simulink model "CrossCorrelator_q"  (R2018b)
settings: Solver=FixedStepAuto  StartTime=0.0  StopTime=500*(15e-9)  FixedStep=15e-9  RelTol=1e-3
libraries: hdlsllib x14, simulink x8
settings Model: Creator=meyer  LastModifiedBy=meyer
settings OptimizationCC: DefaultParameterBehavior=Inlined

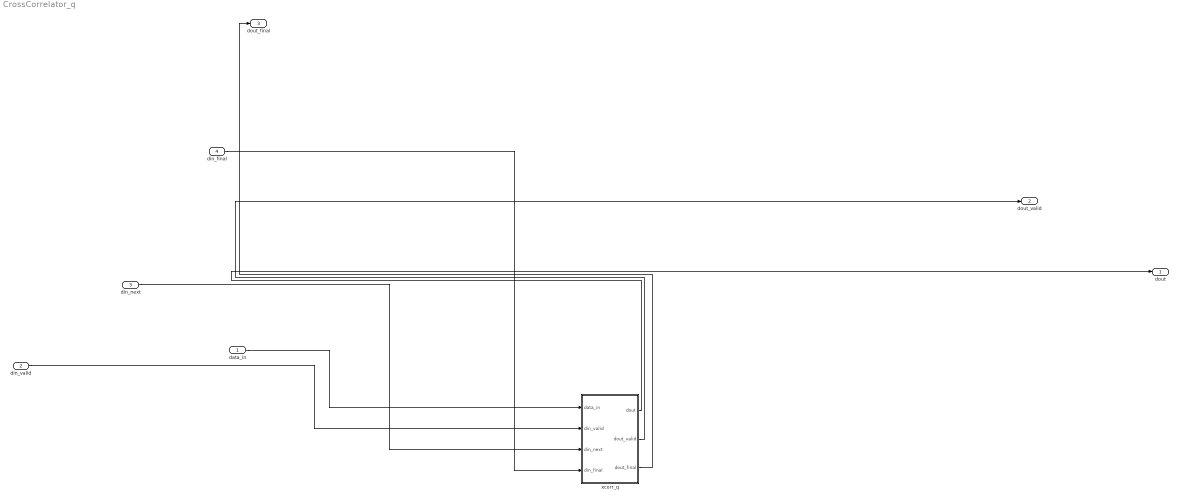
== system CrossCorrelator_q ==
  data_in : Inport  OutDataTypeStr=fixdt(1,16,15)
  din_valid : Inport  Port=2
  din_next : Inport  Port=3
  din_final : Inport  Port=4
  xcorr_q : Subsystem
  dout : Outport  OutDataTypeStr=fixdt(1,32,16)
  dout_valid : Outport  Port=2
  dout_final : Outport  Port=3
  wires:
  data_in/1 -> xcorr_q/1(data_in)
  din_valid/1 -> xcorr_q/2(din_valid)
  din_next/1 -> xcorr_q/3(din_next)
  din_final/1 -> xcorr_q/4(din_final)
  xcorr_q/1(dout) -> dout/1
  xcorr_q/2(dout_valid) -> dout_valid/1
  xcorr_q/3(dout_final) -> dout_final/1

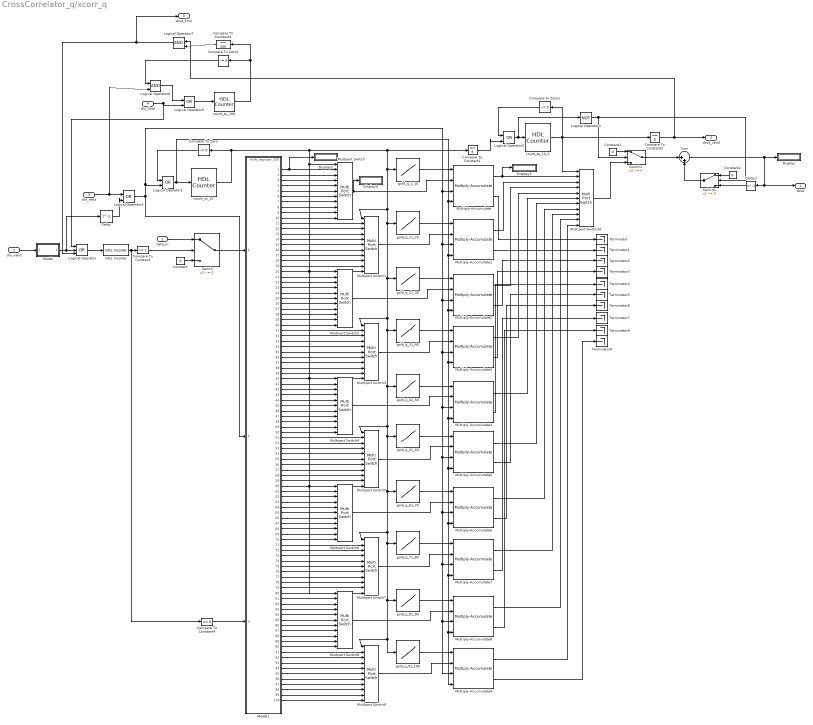
== system CrossCorrelator_q/xcorr_q ==
  data_in : Inport  OutDataTypeStr=fixdt(1,16,15)
  din_valid : Inport  Port=2
  din_next : Inport  Port=3
  din_final : Inport  Port=4
  Compare To Constant : simulink/Logic and Bit Operations/Compare To Constant  relop===  const=1  OutDataTypeStr=boolean
  Compare To Constant1 : simulink/Logic and Bit Operations/Compare To Constant  relop===  const=9  OutDataTypeStr=boolean
  Compare To Constant2 : simulink/Logic and Bit Operations/Compare To Constant  relop===  const=9  OutDataTypeStr=boolean
  Compare To Constant3 : simulink/Logic and Bit Operations/Compare To Constant  relop===  const=100  OutDataTypeStr=boolean
  Compare To Constant4 : simulink/Logic and Bit Operations/Compare To Constant  relop===  const=0  OutDataTypeStr=boolean
  Compare To Zero : simulink/Logic and Bit Operations/Compare To Zero  relop=~=  OutDataTypeStr=boolean
  Compare To Zero1 : simulink/Logic and Bit Operations/Compare To Zero  relop=~=  OutDataTypeStr=boolean
  Compare To Zero2 : simulink/Logic and Bit Operations/Compare To Zero  relop=~=  OutDataTypeStr=boolean
  Constant : Constant  Value=0  OutDataTypeStr=fixdt(1,16,15)  SampleTime=-1
  Constant1 : Constant  Value=0  OutDataTypeStr=Inherit: Inherit via back propagation  SampleTime=-1
  Constant2 : Constant  Value=0  OutDataTypeStr=Inherit: Inherit via back propagation  SampleTime=-1
  Delay : Delay  DelayLength=1
  Delay1 : Delay  DelayLength=1
  Display{,1..3} (4 alike) : Display
  HDL Counter : hdlsllib/Sources/HDL Counter  CountType=Count limited  CountInit=0  CountStep=1  CountMax=2  CountFromType=Initial value  CountFrom=0  CountResetPort=off  CountLoadPort=off  CountEnbPort=on  CountDirPort=off  CountDataType=Unsigned  CountWordLen=8  CountFracLen=0  CountSampTime=1
      settings: SourceProductBaseCode=HD
  Logical Operator : Logic  Operator=OR  Inputs=3  IconShape=distinctive  AllPortsSameDT=off  OutDataTypeStr=boolean
  Logical Operator{1..3,5} (4 alike) : Logic  Operator=OR  IconShape=distinctive  AllPortsSameDT=off  OutDataTypeStr=boolean
  Logical Operator4 : Logic  Operator=NOT  IconShape=distinctive  AllPortsSameDT=off  OutDataTypeStr=boolean
  Logical Operator6 : Logic  IconShape=distinctive  AllPortsSameDT=off  OutDataTypeStr=boolean
  Logical Operator7 : Logic  IconShape=distinctive  AllPortsSameDT=off  OutDataTypeStr=boolean
  Model : ModelReference  ModelNameDialog=re_detect  SimulationMode=Normal  ModelReferenceVersion=1.7
  Model1 : ModelReference  ModelNameDialog=shift_register_100  SimulationMode=Normal  ModelReferenceVersion=1.17
  Multiply-Accumulate{,1..9} (10 alike) : hdlsllib/HDL Operations/Multiply-Accumulate  opMode=Streaming - using Start and End ports  initValueSetting=Dialog  initValue=0  initValueSetting2=Dialog  initValue2=0  initValueSetting3=Dialog  initValue3=0  num_samples=2  RndMeth2=Floor  RndMeth3=Floor  datatype2=fixdt(1,32,16)  datatype3=Inherit: Inherit via back propagation  validOut=on  endInandOut=off  startOut=off  countOut=on  dim=-1  DoSatur=off  parallel=off
      settings: SourceProductName=HDL Coder  SourceProductBaseCode=HD
  Multiport Switch{,1..9} (10 alike) : MultiPortSwitch  DataPortOrder=Zero-based contiguous  Inputs=10  zeroidx=on  OutDataTypeStr=fixdt(1,16,15)
  Multiport Switch10 : MultiPortSwitch  DataPortOrder=Zero-based contiguous  Inputs=10  zeroidx=on  OutDataTypeStr=fixdt(1,32,16)
  Sum : Sum  Inputs=|++  OutDataTypeStr=Inherit: Inherit via back propagation
  Switch : Switch  Criteria=u2 ~= 0  OutDataTypeStr=Inherit: Inherit via back propagation
  Switch1 : Switch  Criteria=u2 ~= 0  OutDataTypeStr=Inherit: Inherit via back propagation
  Switch2 : Switch  Criteria=u2 ~= 0  OutDataTypeStr=Inherit: Inherit via back propagation
  Terminator{,1..9} (10 alike) : Terminator
  count_to_10 : hdlsllib/Sources/HDL Counter  CountType=Count limited  CountInit=0  CountStep=1  CountMax=9  CountFromType=Initial value  CountFrom=0  CountResetPort=off  CountLoadPort=off  CountEnbPort=on  CountDirPort=off  CountDataType=Unsigned  CountWordLen=4  CountFracLen=0  CountSampTime=1
      settings: SourceProductBaseCode=HD
  count_to_100 : hdlsllib/Sources/HDL Counter  CountType=Count limited  CountInit=0  CountStep=1  CountMax=100  CountFromType=Initial value  CountFrom=0  CountResetPort=off  CountLoadPort=off  CountEnbPort=on  CountDirPort=off  CountDataType=Unsigned  CountWordLen=8  CountFracLen=0  CountSampTime=1
      settings: SourceProductBaseCode=HD
  count_to_10_2 : hdlsllib/Sources/HDL Counter  CountType=Count limited  CountInit=0  CountStep=1  CountMax=9  CountFromType=Initial value  CountFrom=0  CountResetPort=off  CountLoadPort=off  CountEnbPort=on  CountDirPort=off  CountDataType=Unsigned  CountWordLen=4  CountFracLen=0  CountSampTime=1
      settings: SourceProductBaseCode=HD
  gold_q_11_20 : Lookup_n-D  NumberOfTableDimensions=1  LookupTableObject=''  BreakpointsForDimension1=uint8([0,1,2,3,4,5,6,7,8,9])  BreakpointsForDimension1FirstPoint=10  BreakpointsForDimension2FirstPoint=10  BreakpointsForDimension1Spacing=12  BreakpointsForDimension2Spacing=12  IndexSearchMethod=Evenly spaced points  Table=|  TableDataTypeStr=fixdt(1,16,15)  InterpMethod=Flat  DiagnosticForOutOfRangeInput=Error  InternalRulePriority=Speed  OutDataTypeStr=fixdt(1,16,15)  RndMeth=Simplest  InputSameDT=on
      | -1*[0.236906374990369
      | 0.265062589296935
      | 0.290853922757751
      | 0.306866645010829
      | 0.306877356493505
      | 0.282583044796408
      | 0.237895318583737
      | 0.179451570247324
      | 0.106711739895776
      | 0.0250742736874029]
  gold_q_1_10 : Lookup_n-D  NumberOfTableDimensions=1  LookupTableObject=''  BreakpointsForDimension1=uint8([0,1,2,3,4,5,6,7,8,9])  BreakpointsForDimension1FirstPoint=10  BreakpointsForDimension2FirstPoint=10  BreakpointsForDimension1Spacing=12  BreakpointsForDimension2Spacing=12  IndexSearchMethod=Evenly spaced points  Table=|  TableDataTypeStr=fixdt(1,16,15)  InterpMethod=Flat  DiagnosticForOutOfRangeInput=Error  InternalRulePriority=Speed  OutDataTypeStr=fixdt(1,16,15)  RndMeth=Simplest  InputSameDT=on
      | -1*[0.357169275362262
      | 0.373691122276015
      | 0.363136475782144
      | 0.332586509539436
      | 0.291374087870011
      | 0.249422279627694
      | 0.215579045674242
      | 0.200455944131647
      | 0.201796906991478
      | 0.213779029408702]
  gold_q_21_30 : Lookup_n-D  NumberOfTableDimensions=1  LookupTableObject=''  BreakpointsForDimension1=uint8([0,1,2,3,4,5,6,7,8,9])  BreakpointsForDimension1FirstPoint=10  BreakpointsForDimension2FirstPoint=10  BreakpointsForDimension1Spacing=12  BreakpointsForDimension2Spacing=12  IndexSearchMethod=Evenly spaced points  Table=|  TableDataTypeStr=fixdt(1,16,15)  InterpMethod=Flat  DiagnosticForOutOfRangeInput=Error  InternalRulePriority=Speed  OutDataTypeStr=fixdt(1,16,15)  RndMeth=Simplest  InputSameDT=on
      | -1*[-0.0591515848508664
      | -0.139598314313151
      | -0.210629837752387
      | -0.263713716480122
      | -0.301489962058033
      | -0.328238114626508
      | -0.340130412877520
      | -0.338689881672749
      | -0.326243180584237
      | -0.305614110780615]
  gold_q_31_40 : Lookup_n-D  NumberOfTableDimensions=1  LookupTableObject=''  BreakpointsForDimension1=uint8([0,1,2,3,4,5,6,7,8,9])  BreakpointsForDimension1FirstPoint=10  BreakpointsForDimension2FirstPoint=10  BreakpointsForDimension1Spacing=12  BreakpointsForDimension2Spacing=12  IndexSearchMethod=Evenly spaced points  Table=|  TableDataTypeStr=fixdt(1,16,15)  InterpMethod=Flat  DiagnosticForOutOfRangeInput=Error  InternalRulePriority=Speed  OutDataTypeStr=fixdt(1,16,15)  RndMeth=Simplest  InputSameDT=on
      | -1*[-0.279858098355888
      | -0.247814863771713
      | -0.225446174923891
      | -0.202743193363060
      | -0.186527042991191
      | -0.178781266249413
      | -0.180711431323688
      | -0.192575241083779
      | -0.213551675353351
      | -0.245925394077466]
  gold_q_41_50 : Lookup_n-D  NumberOfTableDimensions=1  LookupTableObject=''  BreakpointsForDimension1=uint8([0,1,2,3,4,5,6,7,8,9])  BreakpointsForDimension1FirstPoint=10  BreakpointsForDimension2FirstPoint=10  BreakpointsForDimension1Spacing=12  BreakpointsForDimension2Spacing=12  IndexSearchMethod=Evenly spaced points  Table=|  TableDataTypeStr=fixdt(1,16,15)  InterpMethod=Flat  DiagnosticForOutOfRangeInput=Error  InternalRulePriority=Speed  OutDataTypeStr=fixdt(1,16,15)  RndMeth=Simplest  InputSameDT=on
      | -1*[-0.273649789754997
      | -0.305507933389466
      | -0.332526349511340
      | -0.349961882407133
      | -0.353614169955030
      | -0.340366684130075
      | -0.308641627170326
      | -0.254460428744123
      | -0.185247665828561
      | -0.110080691949015]
  gold_q_51_60 : Lookup_n-D  NumberOfTableDimensions=1  LookupTableObject=''  BreakpointsForDimension1=uint8([0,1,2,3,4,5,6,7,8,9])  BreakpointsForDimension1FirstPoint=10  BreakpointsForDimension2FirstPoint=10  BreakpointsForDimension1Spacing=12  BreakpointsForDimension2Spacing=12  IndexSearchMethod=Evenly spaced points  Table=|  TableDataTypeStr=fixdt(1,16,15)  InterpMethod=Flat  DiagnosticForOutOfRangeInput=Error  InternalRulePriority=Speed  OutDataTypeStr=fixdt(1,16,15)  RndMeth=Simplest  InputSameDT=on
      | -1*[-0.0297558495000079
      | 0.0499350486257353
      | 0.122950591883728
      | 0.183532283875116
      | 0.226715241693549
      | 0.244522518247979
      | 0.247772413924009
      | 0.223279362418140
      | 0.176793915855740
      | 0.111355596734925]
  gold_q_61_70 : Lookup_n-D  NumberOfTableDimensions=1  LookupTableObject=''  BreakpointsForDimension1=uint8([0,1,2,3,4,5,6,7,8,9])  BreakpointsForDimension1FirstPoint=10  BreakpointsForDimension2FirstPoint=10  BreakpointsForDimension1Spacing=12  BreakpointsForDimension2Spacing=12  IndexSearchMethod=Evenly spaced points  Table=|  TableDataTypeStr=fixdt(1,16,15)  InterpMethod=Flat  DiagnosticForOutOfRangeInput=Error  InternalRulePriority=Speed  OutDataTypeStr=fixdt(1,16,15)  RndMeth=Simplest  InputSameDT=on
      | -1*[0.0312880626224120
      | -0.0580988665112754
      | -0.150830519884918
      | -0.236354458852815
      | -0.321361371110983
      | -0.387151947785857
      | -0.432910784333285
      | -0.454553321854592
      | -0.449340647995131
      | -0.416266380216616]
  gold_q_71_80 : Lookup_n-D  NumberOfTableDimensions=1  LookupTableObject=''  BreakpointsForDimension1=uint8([0,1,2,3,4,5,6,7,8,9])  BreakpointsForDimension1FirstPoint=10  BreakpointsForDimension2FirstPoint=10  BreakpointsForDimension1Spacing=12  BreakpointsForDimension2Spacing=12  IndexSearchMethod=Evenly spaced points  Table=|  TableDataTypeStr=fixdt(1,16,15)  InterpMethod=Flat  DiagnosticForOutOfRangeInput=Error  InternalRulePriority=Speed  OutDataTypeStr=fixdt(1,16,15)  RndMeth=Simplest  InputSameDT=on
      | -1*[-0.356405677154333
      | -0.268905527196357
      | -0.172503144328213
      | -0.0623088722264564
      | 0.0478292512438748
      | 0.147701871156711
      | 0.227579808283800
      | 0.279365016179912
      | 0.297653875710056
      | 0.276310228166542]
  gold_q_81_90 : Lookup_n-D  NumberOfTableDimensions=1  LookupTableObject=''  BreakpointsForDimension1=uint8([0,1,2,3,4,5,6,7,8,9])  BreakpointsForDimension1FirstPoint=10  BreakpointsForDimension2FirstPoint=10  BreakpointsForDimension1Spacing=12  BreakpointsForDimension2Spacing=12  IndexSearchMethod=Evenly spaced points  Table=|  TableDataTypeStr=fixdt(1,16,15)  InterpMethod=Flat  DiagnosticForOutOfRangeInput=Error  InternalRulePriority=Speed  OutDataTypeStr=fixdt(1,16,15)  RndMeth=Simplest  InputSameDT=on
      | -1*[0.222595237130309
      | 0.147485843722747
      | 0.0555170073150737
      | -0.0424496465550990
      | -0.134707118174198
      | -0.210100315272752
      | -0.259403813850479
      | -0.272248751146779
      | -0.259403813850479
      | -0.210100315272752]
  gold_q_91_100 : Lookup_n-D  NumberOfTableDimensions=1  LookupTableObject=''  BreakpointsForDimension1=uint8([0,1,2,3,4,5,6,7,8,9])  BreakpointsForDimension1FirstPoint=10  BreakpointsForDimension2FirstPoint=10  BreakpointsForDimension1Spacing=12  BreakpointsForDimension2Spacing=12  IndexSearchMethod=Evenly spaced points  Table=|  TableDataTypeStr=fixdt(1,16,15)  InterpMethod=Flat  DiagnosticForOutOfRangeInput=Error  InternalRulePriority=Speed  OutDataTypeStr=fixdt(1,16,15)  RndMeth=Simplest  InputSameDT=on
      | -1*[-0.134707118174198
      | -0.0424496465550989
      | 0.0555170073150737
      | 0.147485843722747
      | 0.222595237130309
      | 0.267820298855522
      | 0.290378842162360
      | 0.275261187855880
      | 0.228204197191429
      | 0.153805243290024]
  dout : Outport  OutDataTypeStr=fixdt(1,32,16)
  dout_valid : Outport  Port=2
  dout_final : Outport  Port=3
  wires:
  Model1/63 -> Multiport Switch6/4
  Model1/83 -> Multiport Switch8/4
  Model1/87 -> Multiport Switch8/8
  Model1/57 -> Multiport Switch5/8
  count_to_10/1 -> Compare To Zero/1, Multiport Switch8/1, Multiport Switch6/1, Multiport Switch4/1, Multiport Switch2/1, Multiport Switch/1, gold_q_11_20/1, gold_q_21_30/1, gold_q_31_40/1, gold_q_41_50/1, gold_q_51_60/1, gold_q_61_70/1, gold_q_71_80/1, gold_q_81_90/1, gold_q_91_100/1, Multiport Switch9/1, Multiport Switch7/1, Multiport Switch5/1, Multiport Switch3/1, Multiport Switch1/1, gold_q_1_10/1, Compare To Constant1/1
  Model1/97 -> Multiport Switch9/8
  Multiply-Accumulate4/1 -> Multiport Switch10/6
  Model1/65 -> Multiport Switch6/6
  Model1/99 -> Multiport Switch9/10
  Model1/73 -> Multiport Switch7/4
  Model1/49 -> Multiport Switch4/10
  Multiply-Accumulate/2 -> Terminator/1
  din_final/1 -> Logical Operator/1, Logical Operator5/2
  count_to_10_2/1 -> Compare To Constant2/1, Multiport Switch10/1, Compare To Zero1/1
  Multiport Switch8/1 -> Multiply-Accumulate8/2
  Compare To Constant2/1 -> dout_valid/1, Logical Operator7/1
  Model1/61 -> Multiport Switch6/2
  Model1/28 -> Multiport Switch2/9
  Model1/1 -> Display2/1, Multiport Switch/2
  Multiply-Accumulate6/1 -> Multiport Switch10/8
  Model1/100 -> Multiport Switch9/11
  Logical Operator/1 -> HDL Counter/1
  din_valid/1 -> Model/1
  Model1/68 -> Multiport Switch6/9
  Model1/56 -> Multiport Switch5/7
  Model1/13 -> Multiport Switch1/4
  Model1/67 -> Multiport Switch6/8
  Model1/66 -> Multiport Switch6/7
  Logical Operator2/1 -> Logical Operator4/1, count_to_10_2/1
  Constant/1 -> Switch/3
  Compare To Zero/1 -> Logical Operator1/1
  Model1/89 -> Multiport Switch8/10
  Multiport Switch5/1 -> Multiply-Accumulate5/2
  Model1/29 -> Multiport Switch2/10
  Compare To Constant/1 -> Switch/2
  gold_q_91_100/1 -> Multiply-Accumulate9/1
  Model1/52 -> Multiport Switch5/3
  Model/1 -> Delay/1, Logical Operator/2
  Logical Operator1/1 -> count_to_10/1, Multiply-Accumulate2/4, Multiply-Accumulate9/4, Multiply-Accumulate8/4, Multiply-Accumulate7/4, Multiply-Accumulate6/4, Multiply-Accumulate5/4, Multiply-Accumulate4/4, Multiply-Accumulate3/4, Multiply-Accumulate1/4, Multiply-Accumulate/4
  Model1/76 -> Multiport Switch7/7
  Sum/1 -> dout/1, Delay1/1, Display/1
  Logical Operator3/1 -> Multiply-Accumulate9/3, Multiply-Accumulate8/3, Multiply-Accumulate7/3, Multiply-Accumulate6/3, Multiply-Accumulate5/3, Multiply-Accumulate4/3, Multiply-Accumulate3/3, Multiply-Accumulate2/3, Multiply-Accumulate1/3, Multiply-Accumulate/3, Logical Operator1/2, Model1/2
  Model1/2 -> Multiport Switch/3
  Model1/88 -> Multiport Switch8/9
  Model1/64 -> Multiport Switch6/5
  Model1/41 -> Multiport Switch4/2
  Multiply-Accumulate9/2 -> Terminator9/1
  din_next/1 -> Logical Operator6/2, Logical Operator3/1
  Model1/11 -> Multiport Switch1/2
  Model1/96 -> Multiport Switch9/7
  Switch1/1 -> Sum/1
  Model1/80 -> Multiport Switch7/11
  Model1/54 -> Multiport Switch5/5
  Model1/82 -> Multiport Switch8/3
  Multiply-Accumulate4/2 -> Terminator4/1
  Model1/6 -> Multiport Switch/7
  Model1/45 -> Multiport Switch4/6
  Multiport Switch4/1 -> Multiply-Accumulate4/2
  Logical Operator4/1 -> Switch1/2, Switch2/2
  Model1/58 -> Multiport Switch5/9
  Model1/81 -> Multiport Switch8/2
  Model1/44 -> Multiport Switch4/5
  Model1/86 -> Multiport Switch8/7
  Model1/85 -> Multiport Switch8/6
  Logical Operator5/1 -> count_to_100/1
  Multiport Switch/1 -> Multiply-Accumulate/2, Display3/1
  Model1/27 -> Multiport Switch2/8
  gold_q_31_40/1 -> Multiply-Accumulate3/1
  Model1/93 -> Multiport Switch9/4
  Compare To Zero1/1 -> Logical Operator2/1
  Model1/39 -> Multiport Switch3/10
  Model1/84 -> Multiport Switch8/5
  Model1/70 -> Multiport Switch6/11
  Model1/77 -> Multiport Switch7/8
  Model1/62 -> Multiport Switch6/3
  Model1/95 -> Multiport Switch9/6
  gold_q_1_10/1 -> Multiply-Accumulate/1
  Compare To Zero2/1 -> Logical Operator6/1
  Multiply-Accumulate1/1 -> Multiport Switch10/3
  Model1/47 -> Multiport Switch4/8
  Multiply-Accumulate3/2 -> Terminator3/1
  Model1/22 -> Multiport Switch2/3
  Model1/92 -> Multiport Switch9/3
  count_to_100/1 -> Compare To Constant3/1, Compare To Zero2/1
  Multiport Switch3/1 -> Multiply-Accumulate3/2
  Model1/59 -> Multiport Switch5/10
  Model1/9 -> Multiport Switch/10
  Model1/5 -> Multiport Switch/6
  gold_q_11_20/1 -> Multiply-Accumulate1/1
  data_in/1 -> Switch/1
  Model1/90 -> Multiport Switch8/11
  Model1/10 -> Multiport Switch/11
  Model1/75 -> Multiport Switch7/6
  Model1/18 -> Multiport Switch1/9
  Model1/12 -> Multiport Switch1/3
  Model1/25 -> Multiport Switch2/6
  Model1/43 -> Multiport Switch4/4
  Model1/72 -> Multiport Switch7/3
  Model1/30 -> Multiport Switch2/11
  Model1/8 -> Multiport Switch/9
  Model1/60 -> Multiport Switch5/11
  HDL Counter/1 -> Compare To Constant4/1, Compare To Constant/1
  Multiply-Accumulate8/2 -> Terminator8/1
  Model1/17 -> Multiport Switch1/8
  Multiply-Accumulate9/1 -> Multiport Switch10/11
  Model1/26 -> Multiport Switch2/7
  Model1/35 -> Multiport Switch3/6
  Model1/24 -> Multiport Switch2/5
  Model1/20 -> Multiport Switch1/11
  Model1/71 -> Multiport Switch7/2
  Model1/78 -> Multiport Switch7/9
  Multiport Switch9/1 -> Multiply-Accumulate9/2
  Model1/7 -> Multiport Switch/8
  Model1/3 -> Multiport Switch/4
  Model1/79 -> Multiport Switch7/10
  Multiport Switch10/1 -> Switch1/3
  Model1/15 -> Multiport Switch1/6
  Model1/14 -> Multiport Switch1/5
  Multiply-Accumulate/1 -> Display1/1, Multiport Switch10/2
  Model1/42 -> Multiport Switch4/3
  Model1/16 -> Multiport Switch1/7
  Logical Operator6/1 -> Logical Operator5/1
  Logical Operator7/1 -> dout_final/1, Logical Operator/3
  Model1/53 -> Multiport Switch5/4
  Model1/37 -> Multiport Switch3/8
  Model1/55 -> Multiport Switch5/6
  Model1/48 -> Multiport Switch4/9
  Model1/4 -> Multiport Switch/5
  Model1/50 -> Multiport Switch4/11
  Model1/40 -> Multiport Switch3/11
  Switch/1 -> Model1/1
  Model1/19 -> Multiport Switch1/10
  Model1/38 -> Multiport Switch3/9
  Model1/33 -> Multiport Switch3/4
  Model1/46 -> Multiport Switch4/7
  Model1/31 -> Multiport Switch3/2
  Model1/69 -> Multiport Switch6/10
  Model1/94 -> Multiport Switch9/5
  gold_q_71_80/1 -> Multiply-Accumulate7/1
  Model1/32 -> Multiport Switch3/3
  Multiply-Accumulate3/1 -> Multiport Switch10/5
  Model1/23 -> Multiport Switch2/4
  Multiply-Accumulate2/1 -> Multiport Switch10/4
  Multiport Switch6/1 -> Multiply-Accumulate6/2
  Constant1/1 -> Switch1/1
  Multiply-Accumulate6/2 -> Terminator6/1
  Compare To Constant1/1 -> Logical Operator2/2
  Constant2/1 -> Switch2/1
  Compare To Constant3/1 -> Logical Operator7/2
  gold_q_41_50/1 -> Multiply-Accumulate4/1
  gold_q_21_30/1 -> Multiply-Accumulate2/1
  Multiport Switch2/1 -> Multiply-Accumulate2/2
  Model1/21 -> Multiport Switch2/2
  gold_q_61_70/1 -> Multiply-Accumulate6/1
  gold_q_51_60/1 -> Multiply-Accumulate5/1
  Multiply-Accumulate7/1 -> Multiport Switch10/9
  Multiport Switch7/1 -> Multiply-Accumulate7/2
  gold_q_81_90/1 -> Multiply-Accumulate8/1
  Multiport Switch1/1 -> Multiply-Accumulate1/2
  Model1/91 -> Multiport Switch9/2
  Multiply-Accumulate5/1 -> Multiport Switch10/7
  Multiply-Accumulate8/1 -> Multiport Switch10/10
  Delay/1 -> Logical Operator3/2
  Delay1/1 -> Switch2/3
  Switch2/1 -> Sum/2
  Model1/51 -> Multiport Switch5/2
  Model1/36 -> Multiport Switch3/7
  Model1/34 -> Multiport Switch3/5
  Compare To Constant4/1 -> Model1/3
  Model1/98 -> Multiport Switch9/9
  Multiply-Accumulate5/2 -> Terminator5/1
  Model1/74 -> Multiport Switch7/5
  Multiply-Accumulate7/2 -> Terminator7/1
  Multiply-Accumulate1/2 -> Terminator1/1
  Multiply-Accumulate2/2 -> Terminator2/1
